simulink model "TestBench"  (Simulink 7.6)
settings: Solver=ode45  StartTime=0.0  StopTime=100  RelTol=1e-3
InitFcn:
  | TestBench_datastruct
  | SCAP
undefined symbols (not defined in the file): determiningBonds, sigbuilder_block
(part 2 of 2)

== system TestBench/TestBenches/V_EngISGTest_experiments/EngineISG/Diesel_Engine/Diesel_Engine/DE_BearingLoss/Computing R ==
  In1 : Inport
  R : Inport  Port=2
  JuncDB : Inport  Port=3
  Bond : Inport  Port=4
  Junction Type : Inport  Port=5
  CalcCausality : Fcn  Expr=(u(1) == u(2) && u(3) ==1) || (u(1) !=u(2) && u(3) == 0)
  CalcOutput : Fcn  Expr=(u(1)*u(2)^u(3))
  MinusOne : Constant  Value=-1
  Mux1 : Mux  Inputs=3
  Mux2 : Mux  Inputs=3
  One : Constant
  Switch1 : MultiPortSwitch  DataPortOrder=Zero-based contiguous  Inputs=2  zeroidx=on  SaturateOnIntegerOverflow=on  InputSameDT=on
  Out1 : Outport
  wires:
  In1/1 -> Mux2/1
  R/1 -> Mux2/2
  JuncDB/1 -> Mux1/1
  Bond/1 -> Mux1/2
  Junction Type/1 -> Mux1/3
  Mux1/1 -> CalcCausality/1
  CalcCausality/1 -> Switch1/1
  One/1 -> Switch1/2
  MinusOne/1 -> Switch1/3
  Switch1/1 -> Mux2/3
  Mux2/1 -> CalcOutput/1
  CalcOutput/1 -> Out1/1

== system TestBench/TestBenches/V_EngISGTest_experiments/EngineISG/ISG/ISG_BG/R_ISG_Bearing/Computing R ==
  In1 : Inport
  R : Inport  Port=2
  JuncDB : Inport  Port=3
  Bond : Inport  Port=4
  Junction Type : Inport  Port=5
  CalcCausality : Fcn  Expr=(u(1) == u(2) && u(3) ==1) || (u(1) !=u(2) && u(3) == 0)
  CalcOutput : Fcn  Expr=(u(1)*u(2)^u(3))
  MinusOne : Constant  Value=-1
  Mux1 : Mux  Inputs=3
  Mux2 : Mux  Inputs=3
  One : Constant
  Switch1 : MultiPortSwitch  DataPortOrder=Zero-based contiguous  Inputs=2  zeroidx=on  SaturateOnIntegerOverflow=on  InputSameDT=on
  Out1 : Outport
  wires:
  In1/1 -> Mux2/1
  R/1 -> Mux2/2
  JuncDB/1 -> Mux1/1
  Bond/1 -> Mux1/2
  Junction Type/1 -> Mux1/3
  Mux1/1 -> CalcCausality/1
  CalcCausality/1 -> Switch1/1
  One/1 -> Switch1/2
  MinusOne/1 -> Switch1/3
  Switch1/1 -> Mux2/3
  Mux2/1 -> CalcOutput/1
  CalcOutput/1 -> Out1/1

== system TestBench/TestBenches/V_EngISGTest_experiments/EngineISG/ISG/ISG_BG/R_ISG_Gyrator/Computing R ==
  In1 : Inport
  R : Inport  Port=2
  JuncDB : Inport  Port=3
  Bond : Inport  Port=4
  Junction Type : Inport  Port=5
  CalcCausality : Fcn  Expr=(u(1) == u(2) && u(3) ==1) || (u(1) !=u(2) && u(3) == 0)
  CalcOutput : Fcn  Expr=(u(1)*u(2)^u(3))
  MinusOne : Constant  Value=-1
  Mux1 : Mux  Inputs=3
  Mux2 : Mux  Inputs=3
  One : Constant
  Switch1 : MultiPortSwitch  DataPortOrder=Zero-based contiguous  Inputs=2  zeroidx=on  SaturateOnIntegerOverflow=on  InputSameDT=on
  Out1 : Outport
  wires:
  In1/1 -> Mux2/1
  R/1 -> Mux2/2
  JuncDB/1 -> Mux1/1
  Bond/1 -> Mux1/2
  Junction Type/1 -> Mux1/3
  Mux1/1 -> CalcCausality/1
  CalcCausality/1 -> Switch1/1
  One/1 -> Switch1/2
  MinusOne/1 -> Switch1/3
  Switch1/1 -> Mux2/3
  Mux2/1 -> CalcOutput/1
  CalcOutput/1 -> Out1/1

== matlab function TestBenches/V_EngISGTest_experiments/EngineISG/PowerController/PowerCtrlBG/CtrlTransformer ==
  data: Ratio output double; InpV input double; OutpV input double; Demand input double
function Ratio = CtrlTransformer(InpV, OutpV, Demand)


if(Demand > 0)
  % Use Power
  if(InpV > .5)
      Ratio =  InpV / Demand;
  else
      Ratio = 0;
  end
else
   % Charge Battery
   Ratio = -Demand / OutpV;
end
if Ratio > 10
  Ratio = 10;
end
Demand 
Ratio

== matlab function TestBenches/V_EngISGTest_experiments/EngineISG/Diesel_Engine/Diesel_Engine/TorqueCalculation ==
  data: lTorque output double; MaxPower input double; Throttle input double; wE input double; torqueMax input double; Additional_Load input double
function lTorque = fcn(MaxPower, Throttle, wE, torqueMax, Additional_Load)



%#eml
% Debugging
% torqueMax = 6000;
power = Throttle*MaxPower
%%% -Additional_Load;
localtorque = power/wE;

if localtorque > torqueMax
 lTorque = torqueMax;
else
 lTorque = power/wE;   
end
